simulink subsystem "single_cell"  (R2021a)
settings: Solver=VariableStepAuto  StartTime=0.0  StopTime=10.0  RelTol=1e-3
libraries: fl_lib x7, nesl_utility x6, ee_lib x1
settings Model: Creator=Carlo Edoardo  LastModifiedBy=mirko

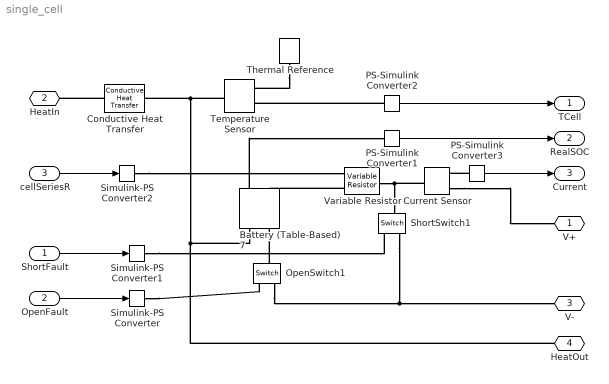
== system single_cell ==
  ShortFault : Inport
  OpenFault : Inport  Port=2
  cellSeriesR : Inport  Port=3
  Battery (Table-Based)7 : ee_lib/Sources/Battery (Table-Based)  Tag={'toolbox/physmod/elec/library/m/ee_lib_parts';'Sources/Battery__Table_Based_/Sanyo/UR18650F.xml'}  SOC_vec=[0 0.01 0.02 0.03 0.04 0.05 0.06 0.07 0.08 0.09 0.1 0.11 0.12 0.13 0.14 0.15 0.16 0.17 0.18 0.19 0.2 0.21 0.22 0.23 0.24 0.25 0.26 0.27 0.28 0.29 0.3 0.31 0.32 0.33 0.34 0.35 0.36 0.37 0.38 0.39 0.4 0.41 0.42 0.43 0.44 0.45 0.46 0.47 0.48 0.49 0.5 0.51 0.52 0.53 0.54 0.55 0.56 0.57 0.58 0.59 0.6 0.61 0.62 0.63 0.64 0.65 0.66 0.67 0.68 0.69 0.7 0.71 0.72 0.73 0.74 0.75 0.76 0.77 0.78 0.79 0.8 0.81 0.82 0.83 0.84 0.85 0.86 0.87 0.88 0.89 0.9 0.91 0.92 0.93 0.94 0.95 0.96 0.97 0.98 0.99 1]  T_dependence=ee.enum.temperature_dependence.yes  prm_dir=ee.enum.battery.prm_dir.noCurrentDirectionality  T_vec=[-20 -10 0 20 40] degC  V0_mat=[3.43105105187538 3.43105105187538 3.43105105187538 3.43105105187538 3.43105105187538;3.58415322083521 3.58415322083521 3.58415322083521 3.58415322083521 3.58415322083521;3.62260441789295 3.62260441789295 3.62260441789295 3.62260441789295 3.62260441789295;3.64734185537851 3.64734185537851 3.64734185537851 3.64734185537851 3.64734185537851;3.64653306426473 3.64653306426473 3.64653306426473 3.64653306426473 3.64653306426473;3.65558876805919 3.65558876805919 3.65558876805919 3.65558876805919 3.65558876805919;3.6633276911556 3.6633276911556 3.6633276911556 3.6633276911556 3.6633276911556;3.66323970812674 3.66323970812674 3.66323970812674 3.66323970812674 3.66323970812674;3.66627838388888 3.66627838388888 3.66627838388888 3.66627838388888 3.66627838388888;3.66945052655532 3.66945052655532 3.66945052655532 3.66945052655532 3.66945052655532;3.67178851675999 3.67178851675999 3.67178851675999 3.67178851675999 3.67178851675999;3.67628180220349 3.67628180220349 3.67628180220349 3.67628180220349 3.67628180220349;3.68207211005278 3.68207211005278 3.68207211005278 3.68207211005278 3.68207211005278;3.68752288461622 3.68752288461622 3.68752288461622 3.68752288461622 3.68752288461622;3.69179433797643 3.69179433797643 3.69179433797643 3.69179433797643 3.69179433797643;3.69629722203264 3.69629722203264 3.69629722203264 3.69629722203264 3.69629722203264;3.70080010608886 3.70080010608886 3.70080010608886 3.70080010608886 3.70080010608886;3.70530299014508 3.70530299014508 3.70530299014508 3.70530299014508 3.70530299014508;3.70960554760222 3.70960554760222 3.70960554760222 3.70960554760222 3.70960554760222;3.71431669425818 3.71431669425818 3.71431669425818 3.71431669425818 3.71431669425818;3.71786846017462 3.71786846017462 3.71786846017462 3.71786846017462 3.71786846017462;3.71960024800499 3.71960024800499 3.71960024800499 3.71960024800499 3.71960024800499;3.72133203583536 3.72133203583536 3.72133203583536 3.72133203583536 3.72133203583536;3.72306382366573 3.72306382366573 3.72306382366573 3.72306382366573 3.72306382366573;3.7247956114961 3.7247956114961 3.7247956114961 3.7247956114961 3.7247956114961;3.72652739932647 3.72652739932647 3.72652739932647 3.72652739932647 3.72652739932647;3.72800897575159 3.72800897575159 3.72800897575159 3.72800897575159 3.72800897575159;3.72938624870664 3.72938624870664 3.72938624870664 3.72938624870664 3.72938624870664;3.73078349806102 3.73078349806102 3.73078349806102 3.73078349806102 3.73078349806102;3.73218074741539 3.73218074741539 3.73218074741539 3.73218074741539 3.73218074741539;3.73400495763149 3.73400495763149 3.73400495763149 3.73400495763149 3.73400495763149;3.73589350831893 3.73589350831893 3.73589350831893 3.73589350831893 3.73589350831893;3.73778205900636 3.73778205900636 3.73778205900636 3.73778205900636 3.73778205900636;3.7396706096938 3.7396706096938 3.7396706096938 3.7396706096938 3.7396706096938;3.74157292813514 3.74157292813514 3.74157292813514 3.74157292813514 3.74157292813514;3.74404252567341 3.74404252567341 3.74404252567341 3.74404252567341 3.74404252567341;3.74672128335847 3.74672128335847 3.74672128335847 3.74672128335847 3.74672128335847;3.74938651767956 3.74938651767956 3.74938651767956 3.74938651767956 3.74938651767956;3.75202648515059 3.75202648515059 3.75202648515059 3.75202648515059 3.75202648515059;3.75466645262162 3.75466645262162 3.75466645262162 3.75466645262162 3.75466645262162;3.75726413936502 3.75726413936502 3.75726413936502 3.75726413936502 3.75726413936502;3.75971222018341 3.75971222018341 3.75971222018341 3.75971222018341 3.75971222018341;3.76216030100179 3.76216030100179 3.76216030100179 3.76216030100179 3.76216030100179;3.76460838182018 3.76460838182018 3.76460838182018 3.76460838182018 3.76460838182018;3.76732650868525 3.76732650868525 3.76732650868525 3.76732650868525 3.76732650868525;3.77045573828492 3.77045573828492 3.77045573828492 3.77045573828492 3.77045573828492;3.77358483833336 3.77358483833336 3.77358483833336 3.77358483833336 3.77358483833336;3.77659854831935 ...(+4548 chars)] V  V0_vec=[3.43105105187538 3.58415322083521 3.62260441789295 3.64734185537851 3.64653306426473 3.65558876805919 3.6633276911556 3.66323970812674 3.66627838388888 3.66945052655532 3.67178851675999 3.67628180220349 3.68207211005278 3.68752288461622 3.69179433797643 3.69629722203264 3.70080010608886 3.70530299014508 3.70960554760222 3.71431669425818 3.71786846017462 3.71960024800499 3.72133203583536 3.72306382366573 3.7247956114961 3.72652739932647 3.72800897575159 3.72938624870664 3.73078349806102 3.73218074741539 3.73400495763149 3.73589350831893 3.73778205900636 3.7396706096938 3.74157292813514 3.74404252567341 3.74672128335847 3.74938651767956 3.75202648515059 3.75466645262162 3.75726413936502 3.75971222018341 3.76216030100179 3.76460838182018 3.76732650868525 3.77045573828492 3.77358483833336 3.77659854831935 3.78019249838402 3.78384910494915 3.78750571151429 3.79116231807942 3.79481892464456 3.79852483410166 3.80289163387691 3.80871318434039 3.81452235122061 3.82033151810084 3.82614068498106 3.83194985186129 3.83775901874152 3.84356818562174 3.84913517632868 3.85462047755666 3.85965250828309 3.86468453900952 3.86971656973595 3.87474860046238 3.88053205579118 3.88655997549109 3.8929556133798 3.89935125126851 3.90676951210798 3.91473885843825 3.92270820476852 3.93067755109879 3.93864689742906 3.94661624375933 3.9545855900896 3.9632866705236 3.97232530006507 3.98134112625335 3.99031265602115 3.99928418578895 4.00825571555675 4.01753782731264 4.02720115749246 4.03686448767229 4.04644536919336 4.05545703375012 4.06446169097151 4.0734663481929 4.08327110755078 4.09372154883564 4.1041719901205 4.11117133518177 4.12181977779421 4.13562611760113 4.14538737309826 4.15501295344536 4.15500359537502] V  R0_mat=[0.406456402801184 0.405110834283117 0.403492406940313 0.325074164245505 0.405354267156167;0.457717348866327 0.431927037644131 0.398282162506819 0.281650920513474 0.25112801914235;0.459130046278384 0.416157375074562 0.354815435766739 0.227074420959134 0.180181420225775;0.45458023952863 0.399877094079194 0.314757287515034 0.18737633452584 0.147072333790223;0.438923376866114 0.379626329437013 0.282279986772266 0.158718545713922 0.13203194617343;0.427555425033268 0.364322097251562 0.256805234861828 0.143607851018012 0.121280469386306;0.420268821916696 0.351184188234578 0.24233040925127 0.132325176131197 0.115599061028902;0.409895460409904 0.335943266376024 0.224452580977545 0.121766449446717 0.107406515272038;0.400881515768766 0.322061761383122 0.212582697956157 0.114671894979549 0.100573386380827;0.391925600216456 0.311139604102015 0.205675227988473 0.110133393647092 0.0961257720153936;0.382607009680764 0.302694518304531 0.198405083037407 0.105663321556782 0.0938577485135764;0.374225504031526 0.295186517393502 0.193137977913942 0.103102948524174 0.092526809898213;0.368429713549107 0.288242439267595 0.189231731778297 0.101691802020488 0.0917597940679712;0.363100340395817 0.281150737973926 0.18517786247489 0.10022848095352 0.0908451550699685;0.357258218893294 0.274516682492735 0.1828711672091 0.0989665029072418 0.0907385023071368;0.351516719432516 0.268671652325336 0.18096011364005 0.097993020996922 0.0912257108494127;0.345775219971738 0.262826622157937 0.179049060071001 0.0970195390866021 0.0917129193916887;0.34003372051096 0.256981591990538 0.177138006501952 0.0960460571762823 0.0922001279339651;0.334205122528848 0.253129236260365 0.175139854411569 0.0950890089492324 0.0926002379549073;0.328554172024479 0.250810393464543 0.173319349798928 0.0947876082763311 0.0931779954535919;0.32524259207934 0.247987472086322 0.171191315140669 0.0944288566068888 0.0932516743698784;0.321359340291691 0.24437325588807 0.16920472560396 0.0935661243149615 0.092534058466134;0.317476088504042 0.240759039689818 0.16721813606725 0.0927033920230337 0.0917894446820305;0.313592836716393 0.237144823491566 0.165231546530541 0.0918406597311064 0.0910037692009125;0.309709584928744 0.233530607293314 0.163244956993831 0.0909779274391786 0.0902180937197938;0.305826333141095 0.230553017062955 0.161258367457121 0.0901151951472513 0.0894324182386756;0.301834293785946 0.228160776106901 0.159162990352913 0.0892729888114563 0.0885379551900579;0.297796905095988 0.225723185816036 0.157022263913894 0.0884158014391626 0.0875981428066299;0.293768201797038 0.223294280916179 0.154890222865883 0.087551146924846 0.0866670158142103;0.289739498498086 0.220865376016322 0.152758181817871 0.0866864924105289 0.0857358888217893;0.2870850527359 0.218622106273735 0.151498592775403 0.0859401548096371 0.0849903969866396;0.284637026283873 0.216406810649123 0.15060073995275 0.085211646866355 0.0842728792694643;0.282188999831846 0.214191515024509 0.149702887130097 0.0844831389230729 0.0835384522577252;0.279740973379819 0.211976219399898 0.148805034307444 0.0837546309797913 0.0827194640821244;0.27729893290775 0.209766909755243 0.14791316746475 0.0830290812242797 0.0819064618864811;0.2751035355213 0.207948165747562 0.147267943707674 0.0827991919460428 0.0813401027764572;0.272999077329108 0.20678154079788 0.146713659144855 0.0827546289878582 0.0808646828606901;0.270888739413452 0.205609036124733 0.146153494858574 0.0827111754114582 0.0803833832214604;0.268767415910814 0.204425545864605 0.145582344985309 0.0826697945873191 0.0798910979952479;0.266646092408175 0.203242055604476 0.145011195112045 0.082628413763179 0.0793988127690345;0.264506385980481 0.202040182419292 0.144421662313725 0.0825779483539839 0.0788881446177664;0.262301633498431 0.200773263179751 0.143767083461049 0.0824953380923447 0.0783124304121415;0.260200260858164 0.199506343940212 0.143096091957456 0.0824127278307065 0.0777367162065187;0.258613731217304 0.198239424700671 0.142408391648729 0.0823301175690673 0.0771771128329189 ...(+5215 chars)] Ohm  R0_vec=[0.325074164245505 0.281650920513474 0.227074420959134 0.18737633452584 0.158718545713922 0.143607851018012 0.132325176131197 0.121766449446717 0.114671894979549 0.110133393647092 0.105663321556782 0.103102948524174 0.101691802020488 0.10022848095352 0.0989665029072418 0.097993020996922 0.0970195390866021 0.0960460571762823 0.0950890089492324 0.0947876082763311 0.0944288566068888 0.0935661243149615 0.0927033920230337 0.0918406597311064 0.0909779274391786 0.0901151951472513 0.0892729888114563 0.0884158014391626 0.087551146924846 0.0866864924105289 0.0859401548096371 0.085211646866355 0.0844831389230729 0.0837546309797913 0.0830290812242797 0.0827991919460428 0.0827546289878582 0.0827111754114582 0.0826697945873191 0.082628413763179 0.0825779483539839 0.0824953380923447 0.0824127278307065 0.0823301175690673 0.0823223408989603 0.0823999095937525 0.0822767028973347 0.0820512548515318 0.0819504792189938 0.08186316618135 0.0817758531437057 0.0816885401060614 0.0816012270684181 0.0815245074226264 0.0815980433835433 0.0819583882500015 0.0823077606441779 0.0826571330383548 0.0830065054325321 0.0833558778267085 0.0837052502208859 0.0840546226150632 0.0844052709489593 0.0847094577998779 0.084612024383608 0.0845145909673381 0.0844171575510677 0.0843197241347982 0.0844305211386789 0.084558733772419 0.0846567808451425 0.0847548279178669 0.0851199133434577 0.0856802640302693 0.0862406147170815 0.0868009654038931 0.0873613160907047 0.0879216667775173 0.0884820174643284 0.0892137880311289 0.090025366119288 0.0908167392993968 0.091568863642079 0.0923209879847611 0.0930731123274438 0.0938332675954455 0.0946040770361837 0.0953748864769204 0.0960726422946134 0.0962715413096597 0.0964684984926431 0.0966654556756264 0.097035135025892 0.0975436539443687 0.0980521728628454 0.0953198505812296 0.0931936709617899 0.0911825563121402 0.0847179508088908 0.0781331303571324 0.0630112740110763] Ohm  R0_dis_mat=[0.03 0.015 0.002;0.04 0.017 0.008;0.039 0.012 0.006;0.027 0.013 0.021] % Parameter not set Ohm  R0_dis_vec=[0.015 0.017 0.012 0.013] % Parameter not set Ohm  R0_ch_mat=[0.03 0.015 0.002;0.04 0.017 0.008;0.039 0.012 0.006;0.027 0.013 0.021] % Parameter not set Ohm  R0_ch_vec=[0.015 0.017 0.012 0.013] % Parameter not set Ohm  AH_vec=[1.81270032971044 2.16619011419561 2.2621229968348 2.37612929889533 2.39597127172487] hr*A  AH=2.37612929889533 hr*A  prm_leak=ee.enum.battery.prm_leak.disabled  Rleak_vec=[8000 7000 6000] % Parameter not set Ohm  Rleak=7000 % Parameter not set Ohm  extrapolation_option=ee.enum.extrapolation.nearest  prm_dyn=ee.enum.battery.prm_dyn.off  R1_mat=[0.089 0.076 0.01;0.042 0.022 0.099;0.019 0.007 0.002;0.051 0.043 0.029] % Parameter not set Ohm  R1_vec=[0.076 0.022 0.007 0.043] % Parameter not set Ohm  tau1_mat=[44 148 235;93 110 1000;19 27 133;0.5 22 3] % Parameter not set s  tau1_vec=[148 110 27 22] % Parameter not set s  R2_mat=[0.014 0.382 0.407;0.028 0.006 0.007;0.014 0.007 0.006;0.333 0.956 0.912] % Parameter not set Ohm  R2_vec=[0.382 0.006 0.007 0.956] % Parameter not set Ohm  tau2_mat=[1 44 5644;11 24 506;2 14 330;3310 13419 30216] % Parameter not set s  tau2_vec=[44 24 14 13419] % Parameter not set s  R3_mat=[0.014 0.382 0.407;0.028 0.006 0.007;0.014 0.007 0.006;0.333 0.956 0.912] % Parameter not set Ohm  R3_vec=[0.382 0.006 0.007 0.956] % Parameter not set Ohm  tau3_mat=[1 44 5644;11 24 506;2 14 330;3310 13419 30216] % Parameter not set s  tau3_vec=[44 24 14 13419] % Parameter not set s  R4_mat=[0.014 0.382 0.407;0.028 0.006 0.007;0.014 0.007 0.006;0.333 0.956 0.912] % Parameter not set Ohm  R4_vec=[0.382 0.006 0.007 0.956] % Parameter not set Ohm  tau4_mat=[1 44 5644;11 24 506;2 14 330;3310 13419 30216] % Parameter not set s  tau4_vec=[44 24 14 13419] % Parameter not set s  R5_mat=[0.014 0.382 0.407;0.028 0.006 0.007;0.014 0.007 0.006;0.333 0.956 0.912] % Parameter not set Ohm  R5_vec=[0.382 0.006 0.007 0.956] % Parameter not set Ohm  tau5_mat=[1 44 5644;11 24 506;2 14 330;3310 13419 30216] % Parameter not set s  tau5_vec=[44 24 14 13419] % Parameter not set s  prm_fade=ee.enum.battery.prm_fade.tableN  N0=100 % Parameter not set  dV0=0 % Parameter not set  dR0=0 % Parameter not set  dAH=0 % Parameter not set  dRleak=0 % Parameter not set  dR1=0 % Parameter not set  dR2=0 % Parameter not set  dR3=0 % Parameter not set  dR4=0 % Parameter not set  dR5=0 % Parameter not set  N0vec=[1 6 11 16 21 26 31 36 41 46 51 56 61 66 71 76 81 86 91 96 101 106 111 116 121 126 131 136 141 146 151 156 161 166 171 176 181 186 191 196 201 206 211 216 221 226 231 236 241 246 251 256 261 266 271 276 281 286 291 296 301 306 311 316 321 326 331 336 341 346 351 356 361 366 371 376 381 386 391 396 401 406 411 416 421 426 431 436 441 446 451 456 461 466 471 476 481 486 491 496]  Tfadevec=[298.15 323.15] % Parameter not set K  dV0vec=[0 0.000111228896491326 0.000222457793025403 -0.111337857344165 -0.225746345534032 -0.341687238659398 -0.457547850881251 -0.529843539153571 -0.605793024803614 -0.681742510453677 -0.75769199610372 -0.825637295268894 -0.88421500309724 -0.942792710925565 -1.00987654375021 -1.07243861764233 -1.11956237899412 -1.16668614034588 -1.21380990169769 -1.27944841665078 -1.34205865042584 -1.40030822017924 -1.45855778993262 -1.516807359686 -1.57505692943941 -1.63330649919279 -1.69155606894617 -1.74836027020817 -1.8030108824229 -1.85766149463761 -1.91231210685234 -1.96648266910772 -2.01636878810109 -2.06625490709447 -2.11614102608785 -2.16602714508122 -2.21591326407458 -2.26579938306795 -2.31568550206131 -2.36557162105466 -2.41547301905012 -2.46539795892883 -2.51532289880751 -2.56524783868622 -2.61532829039498 -2.66840671235715 -2.71987160426858 -2.77078558318733 -2.82169956210603 -2.87286582255724 -2.92421794375589 -2.97557006495456 -3.02692218615321 -3.07827430735188 -3.12962642855055 -3.18097854974922 -3.22804366252926 -3.27219425515625 -3.31603297027245 -3.35844182179939 -3.40085067332632 -3.44325952485326 -3.48566837638018 -3.52807722790712 -3.56919281070042 -3.61018265050181 -3.65117249030321 -3.69216233010461 -3.73695592398304 -3.7827637709751 -3.82857161796716 -3.87437946495921 -3.92018731195125 -3.96599515894331 -4.01180300593535 -4.05761085292739 -4.10341869991944 -4.14922654691148 -4.19444481103074 -4.23752500080704 -4.28060519058331 -4.32368538035961 -4.3667655701359 -4.40987929794346 -4.45306844864724 -4.49625759935102 -4.5394467500548 -4.58263590075857 -4.62538798996279 -4.66696423472703 -4.71162331366988 -4.75648974226807 -4.80135617086626 -4.84431454621232 -4.88540784615516 -4.92650114609798 -4.96759444604083 -5.00868774598367 -5.04978104592653 -5.0908743458694]  dR0vec=[0;0;0;0;0;0;0;0;0;0;0;0;0;0;0;0;0;0;0;0;0;0;0;0;0;0;0;0;0;0;0;0;0;0;0;0;0;0;0;0;0;0;0;0;0;0;0;0;0;0;0;0;0;0;0;0;0;0;0;0;0;0;0;0;0;0;0;0;0;0;0;0;0;0;0;0;0;0;0;0;0;0;0;0;0;0;0;0;0;0;0;0;0;0;0;0;0;0;0;0] % Parameter not set  dAHvec=[0 -0.493858720854541 -0.987717441709062 -1.48157616256358 -1.97543488341812 -2.46929360427265 -2.96246915990247 -3.19103834649066 -3.41960753307886 -3.64817671966707 -3.87674590625527 -4.10531509284348 -4.33388427943168 -4.56245346601989 -4.82421340286948 -5.10395300154653 -5.38369260022356 -5.66343219890059 -5.94317179757763 -6.22291139625468 -6.47184418229843 -6.70343935149474 -6.93503452069106 -7.16662968988738 -7.39822485908369 -7.62982002828001 -7.86141519747632 -8.09301036667264 -8.32460553586896 -8.55620070506527 -8.78779587426159 -9.01889893391268 -9.24908760037772 -9.47927626684277 -9.70946493330783 -9.93965359977288 -10.1698422662379 -10.400030932703 -10.630219599168 -10.8604082656331 -11.0905969320981 -11.3207855985632 -11.5509742650282 -11.7811629314933 -12.0113515979583 -12.2415402644234 -12.4647314295132 -12.6855334141706 -12.9063353988281 -13.1271373834855 -13.347939368143 -13.5687413528004 -13.7895433374579 -14.0103453221153 -14.2311473067728 -14.4519492914302 -14.6543181530738 -14.8441552668734 -15.0339923806729 -15.2238294944725 -15.413666608272 -15.6035037220716 -15.7933408358712 -15.9831779496707 -16.1730150634703 -16.3628521772699 -16.5526892910694 -16.742526404869 -16.9499799255412 -17.1621307781544 -17.3742816307675 -17.5864324833807 -17.7985833359938 -18.010734188607 -18.2228850412201 -18.4350358938333 -18.6471867464464 -18.8593375990596 -19.0684200837275 -19.2669580098942 -19.4654959360609 -19.6640338622276 -19.8625717883943 -20.0611097145609 -20.2596476407276 -20.4581855668943 -20.656723493061 -20.8552614192277 -21.0537993453944 -21.2523372715611 -21.465596573071 -21.6798460258271 -21.8940954785831 -22.1083449313392 -22.3225943840952 -22.5368438368512 -22.7510932896073 -22.9653427423633 -23.1795921951194 -23.3938416478754]  dRleakvec=[0 0 0] % Parameter not set  dR1vec=[0 0 0] % Parameter not set  dR2vec=[0 0 0] % Parameter not set  dR3vec=[0 0 0] % Parameter not set  dR4vec=[0 0 0] % Parameter not set  dR5vec=[0 0 0] % Parameter not set  dV0mat=[0 0;0 0;0 0] % Parameter not set  dR0mat=[0 0;0 0;0 0] % Parameter not set  dAHmat=[0 0;0 0;0 0] % Parameter not set  dRleakmat=[0 0;0 0;0 0] % Parameter not set  dR1mat=[0 0;0 0;0 0] % Parameter not set  dR2mat=[0 0;0 0;0 0] % Parameter not set  dR3mat=[0 0;0 0;0 0] % Parameter not set  dR4mat=[0 0;0 0;0 0] % Parameter not set  dR5mat=[0 0;0 0;0 0] % Parameter not set  prm_age=ee.enum.battery.prm_age.disabled  prm_age_OCV=ee.enum.battery.prm_age_OCV.SOC  OCV_age=0.9 % Parameter not set  SOC_age=0.6 % Parameter not set  storage_dt_age_vec=0 % Parameter not set d  storage_T_age_vec=273 % Parameter not set K  OCV_scaling_age=2213400 % Parameter not set  OCV_offset_age=1632000 % Parameter not set  temp_exp_age=0.515833569 % Parameter not set V  t_exp_age=0.75 % Parameter not set  T_age_vec=[273.15 298.15 323.15] % Parameter not set K  dt_age_vec=[90 180 270 360] % Parameter not set d  dR0_age_vec=[0 0 0] % Parameter not set  t_meas_dR0_age=100 % Parameter not set d  dR0_age_mat=[0 0 0;0 0 0;0 0 0;0 0 0] % Parameter not set  temperature=298.15 K  i_specify=off  i_priority=None  i=0 A  i_nominal_specify=off  i_nominal_unit=A  i_nominal_value=1  v_specify=off  v_priority=None  v=0 V  v_nominal_specify=off  v_nominal_unit=V  v_nominal_value=1  stateOfCharge_specify=on  stateOfCharge_priority=High  stateOfCharge=1  stateOfCharge_nominal_specify=off  stateOfCharge_nominal_unit=1  stateOfCharge_nominal_value=1  num_cycles_specify=off  num_cycles_priority=High  num_cycles=0  num_cycles_nominal_specify=off  num_cycles_nominal_unit=1  num_cycles_nominal_value=1  thermal_mass=CellThermalMass J/K  temperature_specify=on  temperature_priority=High  temperature_nominal_specify=off  temperature_nominal_unit=K  temperature_nominal_value=1
      settings: AttributesFormatString=Sanyo:UR18650F  SourceProductBaseCode=PS  InternalSimscapePortConfiguration="{\"Bottom\":[],\"Left\":[{\"id\":\"p\",\"label\":\"+\",\"type\":\"foundation.electrical.electrical\"},{\"id\":\"soc\",\"label\":\"SOC\",\"type\":\"output\"}],\"Right\":[{\"id\":\"n\",\"label\":\"-\",\"type\":\"foundation.electrical.electrical\"},{\"id\":\"H\",\"label\":\"H\",\"type\":\"foundation.thermal.thermal\"}],\"Top\":[]}"
  Conductive Heat Transfer : fl_lib/Thermal/Thermal Elements/Conductive Heat Transfer  area=Cell2CellConductiveArea m^2  thickness=Cell2CellConductiveThickness mm  th_cond=Cell2CellConductiveThermConduct W/(m*K)  T_specify=off  T_priority=None  T=0 K  T_nominal_specify=off  T_nominal_unit=K  T_nominal_value=1  Q_specify=off  Q_priority=None  Q=0 W  Q_nominal_specify=off  Q_nominal_unit=W  Q_nominal_value=1
  Current Sensor : fl_lib/Electrical/Electrical Sensors/Current Sensor
  OpenSwitch1 : fl_lib/Electrical/Electrical Elements/Switch  R_closed=1e-12 Ohm  G_open=1e-10 1/Ohm  Threshold=0.5  i_specify=off  i_priority=None  i=0 A  i_nominal_specify=off  i_nominal_unit=A  i_nominal_value=1  v_specify=off  v_priority=None  v=0 V  v_nominal_specify=off  v_nominal_unit=V  v_nominal_value=1
  PS-Simulink Converter1 : nesl_utility/PS-Simulink Converter  PhysicalDomain=network_engine_domain  SubClassName=ps_output  LeftPortType=input  RightPortType=output  PseudoPeriodic=off  Frequencies=[]  Unit=inherit  AffineConversion=off
      settings: SourceProductBaseCode=PW,SS
  PS-Simulink Converter2 : nesl_utility/PS-Simulink Converter  PhysicalDomain=network_engine_domain  SubClassName=ps_output  LeftPortType=input  RightPortType=output  PseudoPeriodic=off  Frequencies=[]  Unit=inherit  AffineConversion=off
      settings: SourceProductBaseCode=PW,SS
  PS-Simulink Converter3 : nesl_utility/PS-Simulink Converter  PhysicalDomain=network_engine_domain  SubClassName=ps_output  LeftPortType=input  RightPortType=output  PseudoPeriodic=off  Frequencies=[]  Unit=inherit  AffineConversion=off
      settings: SourceProductBaseCode=PW,SS
  ShortSwitch1 : fl_lib/Electrical/Electrical Elements/Switch  R_closed=1e-10 Ohm  G_open=1e-10 1/Ohm  Threshold=0.5  i_specify=off  i_priority=None  i=0 A  i_nominal_specify=off  i_nominal_unit=A  i_nominal_value=1  v_specify=off  v_priority=None  v=0 V  v_nominal_specify=off  v_nominal_unit=V  v_nominal_value=1
  Simulink-PS Converter : nesl_utility/Simulink-PS Converter  PhysicalDomain=network_engine_domain  SubClassName=ps_input  LeftPortType=input  RightPortType=output  PseudoPeriodic=off  Frequencies=[]  NoiseDistribution=none  NoiseParameters=[]  Unit=1  AffineConversion=off  FilteringAndDerivatives=provide  SimscapeFilterOrder=1  InputFilterTimeConstant=0.001  UdotUserProvided=0
      settings: SourceProductBaseCode=PW,SS
  Simulink-PS Converter1 : nesl_utility/Simulink-PS Converter  PhysicalDomain=network_engine_domain  SubClassName=ps_input  LeftPortType=input  RightPortType=output  PseudoPeriodic=off  Frequencies=[]  NoiseDistribution=none  NoiseParameters=[]  Unit=1  AffineConversion=off  FilteringAndDerivatives=provide  SimscapeFilterOrder=1  InputFilterTimeConstant=0.001  UdotUserProvided=0
      settings: SourceProductBaseCode=PW,SS
  Simulink-PS Converter2 : nesl_utility/Simulink-PS Converter  PhysicalDomain=network_engine_domain  SubClassName=ps_input  LeftPortType=input  RightPortType=output  PseudoPeriodic=off  Frequencies=[]  NoiseDistribution=none  NoiseParameters=[]  Unit=1  AffineConversion=off  FilteringAndDerivatives=provide  SimscapeFilterOrder=1  InputFilterTimeConstant=0.001  UdotUserProvided=0
      settings: SourceProductBaseCode=PW,SS
  Temperature Sensor : fl_lib/Thermal/Thermal Sensors/Temperature Sensor
  Thermal Reference : fl_lib/Thermal/Thermal Elements/Thermal Reference
  Variable Resistor : fl_lib/Electrical/Electrical Elements/Variable Resistor  Rmin=0 Ohm  i_specify=off  i_priority=None  i=0 A  i_nominal_specify=off  i_nominal_unit=A  i_nominal_value=1  v_specify=off  v_priority=None  v=0 V  v_nominal_specify=off  v_nominal_unit=V  v_nominal_value=1
  V+ : PMIOPort  Side=Right
  HeatIn : PMIOPort  Port=2  Side=Left
  V- : PMIOPort  Port=3  Side=Right
  HeatOut : PMIOPort  Port=4  Side=Left
  TCell : Outport
  RealSOC : Outport  Port=2
  Current : Outport  Port=3
  wires:
  ShortFault/1 -> Simulink-PS Converter1/1
  OpenFault/1 -> Simulink-PS Converter/1
  PS-Simulink Converter2/1 -> TCell/1
  PS-Simulink Converter1/1 -> RealSOC/1
  cellSeriesR/1 -> Simulink-PS Converter2/1
  PS-Simulink Converter3/1 -> Current/1
  connections:
  Temperature Sensor/LConn1 -- Battery (Table-Based)7/RConn2 -- HeatOut/RConn1 -- Conductive Heat Transfer/RConn1
  OpenSwitch1/RConn2 -- V-/RConn1 -- ShortSwitch1/RConn2
  Variable Resistor/RConn1 -- ShortSwitch1/LConn1 -- Current Sensor/LConn1
  Simulink-PS Converter1/RConn1 -- ShortSwitch1/RConn1
  Battery (Table-Based)7/LConn2 -- PS-Simulink Converter1/LConn1
  Thermal Reference/LConn1 -- Temperature Sensor/RConn1
  PS-Simulink Converter2/LConn1 -- Temperature Sensor/RConn2
  Simulink-PS Converter/RConn1 -- OpenSwitch1/RConn1
  OpenSwitch1/LConn1 -- Battery (Table-Based)7/RConn1
  Conductive Heat Transfer/LConn1 -- HeatIn/RConn1
  Variable Resistor/LConn2 -- Battery (Table-Based)7/LConn1
  Simulink-PS Converter2/RConn1 -- Variable Resistor/LConn1
  Current Sensor/RConn2 -- V+/RConn1
  PS-Simulink Converter3/LConn1 -- Current Sensor/RConn1
